simulink model "apf"  (R2025b)
settings: Solver=ode1  StartTime=0.0  StopTime=25  FixedStep=0.05  RelTol=1e-3
libraries: robotcorelib x1
settings Model: Creator=haider  LastModifiedBy=haider

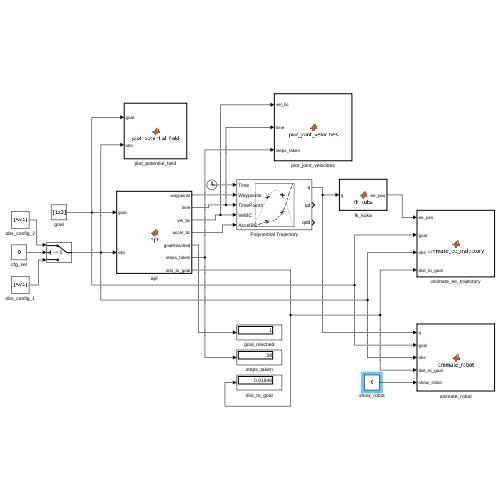
[thumbnail: Simulink's stored preview of the top-level diagram]
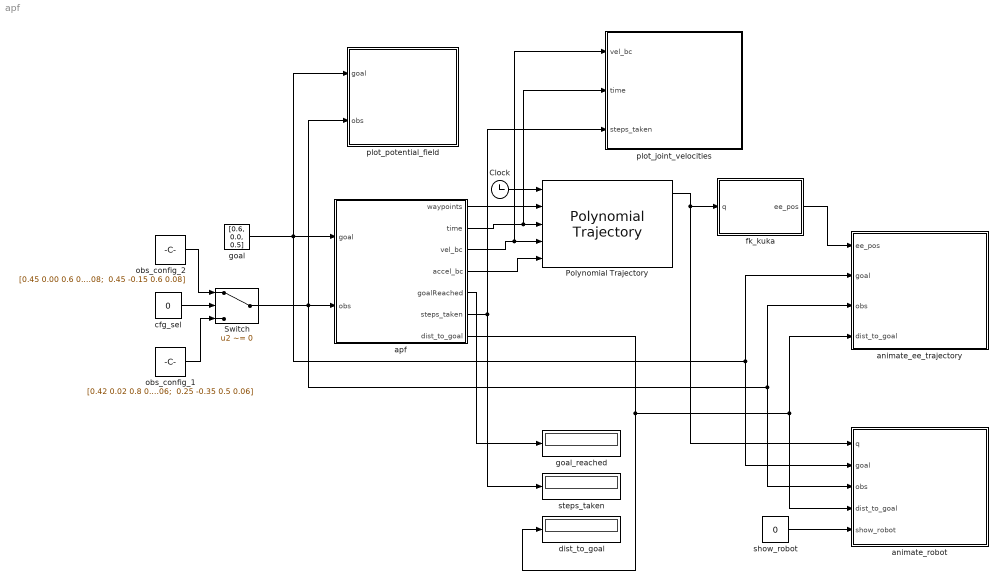
== system apf ==
  Clock : Clock
  Polynomial Trajectory : robotcorelib/Polynomial Trajectory  WaypointSource=External  Waypoints=[ 0, 2, 1, 5, 0; -1, 3, 1, 4, 4 ]  TimePoints=[ 0, 1, 2, 3, 4 ]  TimeInterval=[ 1, 4 ]  Method=Quintic Polynomial  ParameterSource=External  VelocityBoundaryCondition=zeros( 2, 5 )  AccelerationBoundaryCondition=zeros( 2, 5 )  SimulateUsing=Interpreted execution
  Switch : Switch  Criteria=u2 ~= 0  SaturateOnIntegerOverflow=off  InputSameDT=off
  animate_ee_trajectory : MATLAB Function  TreatAsAtomicUnit=on
  animate_robot : MATLAB Function  TreatAsAtomicUnit=on
  apf : MATLAB Function  TreatAsAtomicUnit=on
  cfg_sel : Constant  Value=0
  dist_to_goal : Display
  fk_kuka : MATLAB Function  TreatAsAtomicUnit=on
  goal : Constant  Value=[0.6, 0.0, 0.5]  VectorParams1D=off
  goal_reached : Display
  obs_config_1 : Constant  Value=|  VectorParams1D=off
      | [0.42 0.02 0.8 0.06;
      |  0.45 -0.10 0.4 0.06;
      |  0.35 0.15 0.7 0.06;
      |  0.55 0.30 0.4 0.06;
      |  0.25 -0.35 0.5 0.06]
  obs_config_2 : Constant  Value=|  VectorParams1D=off
      | [0.45 0.00 0.6 0.08;
      |  0.35 0.15 0.6 0.08;
      |  0.45 0.15 0.6 0.08;
      |  0.35 -0.15 0.6 0.08;
      |  0.45 -0.15 0.6 0.08]
  plot_joint_velocities : MATLAB Function  TreatAsAtomicUnit=on
  plot_potential_field : MATLAB Function  TreatAsAtomicUnit=on
  show_robot : Constant  Value=0
  steps_taken : Display
  wires:
  goal/1 -> plot_potential_field/1(goal), animate_robot/2(goal), animate_ee_trajectory/2(goal), apf/1(goal)
  Switch/1 -> animate_robot/3(obs), animate_ee_trajectory/3(obs), plot_potential_field/2(obs), apf/2(obs)
  cfg_sel/1 -> Switch/2
  obs_config_2/1 -> Switch/1
  obs_config_1/1 -> Switch/3
  Clock/1 -> Polynomial Trajectory/1
  apf/1(waypoints) -> Polynomial Trajectory/2
  apf/2(time) -> Polynomial Trajectory/3, plot_joint_velocities/2(time)
  apf/3(vel_bc) -> plot_joint_velocities/1(vel_bc), Polynomial Trajectory/4
  apf/4(accel_bc) -> Polynomial Trajectory/5
  Polynomial Trajectory/1 -> fk_kuka/1(q), animate_robot/1(q)
  fk_kuka/1(ee_pos) -> animate_ee_trajectory/1(ee_pos)
  apf/7(dist_to_goal) -> dist_to_goal/1, animate_robot/4(dist_to_goal), animate_ee_trajectory/4(dist_to_goal)
  show_robot/1 -> animate_robot/5(show_robot)
  apf/6(steps_taken) -> steps_taken/1, plot_joint_velocities/3(steps_taken)
  apf/5(goalReached) -> goal_reached/1

== matlab function apf/plot_potential_field ==
  data: goal input; obs input
function plot_potential_field(goal, obs)
%#codegen

persistent fig_created;

if isempty(fig_created)
    fig_created = false;
end

k_att  = 4.0;
k_rep  = 0.04;
d_star = 0.3;
rho_0  = 0.05;

res     = 100;
x_range = linspace(-0.5, 1.0, res);
y_range = linspace(-0.5, 1.0, res);

z_slice = goal(3);

[X, Y] = meshgrid(x_range, y_range);

U_total = zeros(res, res);

for xi = 1:res
    for yi = 1:res

        p = [X(yi,xi), Y(yi,xi), z_slice];

        % Attractive potential
        rho_att = norm(p - goal);

        if rho_att <= d_star
            U_att = 0.5 * k_att * rho_att^2;
        else
            U_att = d_star * k_att * rho_att ...
                  - 0.5 * k_att * d_star^2;
        end

        % Repulsive potential
        U_rep = 0;

        for j = 1:size(obs,1)

            obs_p = obs(j,1:3);
            obs_r = obs(j,4);

            rho = norm(p - obs_p) - obs_r;

            if rho <= rho_0 && rho > 0.001
                U_rep = U_rep + ...
                    0.5 * k_rep * (1/rho - 1/rho_0)^2;
            end

        end

        U_total(yi,xi) = U_att + U_rep;

    end
end

if ~fig_created

    fig_created = true;

    % Clip extreme values for better visualization
    U_plot = min(U_total, prctile(U_total(:),95));

    figure('Visible','on');

    surf(X,Y,U_plot,'EdgeColor','none');

    colormap(gca,jet);
    colorbar;
    hold on;

    % Goal marker
    plot3(goal(1),goal(2),0,...
        'gp',...
        'MarkerSize',15,...
        'MarkerFaceColor','g');

    % Obstacle slice outlines
    for j = 1:size(obs,1)

        obs_p = obs(j,1:3);
        obs_r = obs(j,4);

        dz = abs(obs_p(3) - z_slice);

        if dz < obs_r

            r_slice = sqrt(obs_r^2 - dz^2);

            theta = linspace(0,2*pi,60);

            cx = obs_p(1) + r_slice*cos(theta);
            cy = obs_p(2) + r_slice*sin(theta);

            plot3(cx,cy,zeros(size(cx)),...
                'r-',...
                'LineWidth',2);

        end

    end

    xlabel('X (m)');
    ylabel('Y (m)');
    zlabel('U_{total}');

    title(sprintf( ...
        'APF Potential Landscape (z = %.2f m)', ...
        z_slice));

    view(45,35);
    grid on;

end

end

== matlab function apf/apf ==
  data: goal input; waypoints output; obs input; time output; vel_bc output; accel_bc output; goalReached output; steps_taken output; dist_to_goal output
function [waypoints, time, vel_bc, accel_bc, goalReached, steps_taken, dist_to_goal] = apf(goal, obs)

%#codegen
MAX_ITER = 500;


persistent planned

persistent wp_cache
persistent time_cache
persistent vel_cache
persistent accel_cache
persistent goal_cache
persistent steps_cache
persistent dist_cache

if isempty(planned)

    planned = false;

    wp_cache    = zeros(7,MAX_ITER);
    time_cache  = zeros(1,MAX_ITER);
    vel_cache   = zeros(7,MAX_ITER);
    accel_cache = zeros(7,MAX_ITER);

    goal_cache  = false;
    steps_cache = int32(0);
    dist_cache  = 0;

end

if planned

    waypoints    = wp_cache;
    time         = time_cache;
    vel_bc       = vel_cache;
    accel_bc     = accel_cache;
    goalReached  = goal_cache;
    steps_taken  = steps_cache;
    dist_to_goal = dist_cache;

    return;

end


% Pre-allocate fixed-size outputs with NaN so unused slots are ignored
waypoints = nan(7, MAX_ITER);
vel_bc    = nan(7, MAX_ITER);
accel_bc  = nan(7, MAX_ITER);
time      = zeros(1, MAX_ITER);

goalReached = false;
steps_taken = int32(0);

% APF params
k_att     = 4.0;
k_rep     = 0.04;
dt        = 0.05;
threshold = 0.02;
rho_0     = 0.05;
iterations = MAX_ITER;
d_star    = 0.3;
q_dot_max = 5.0;

ee_body = 'iiwa_link_ee';

collision_links = { ...
    'iiwa_link_4'; ...
    'iiwa_link_5'; ...
    'iiwa_link_6'; ...
    'iiwa_link_ee' ...
};

robot = loadrobot('kukaIiwa14', 'DataFormat', 'row');
q = homeConfiguration(robot);   % 1x7 row vector

goal = goal(:)';

pos_buffer = zeros(3, 15);
q_dot_prev = zeros(1,7);

for i = 1:iterations

    % Forward kinematics
    T_ee = getTransform(robot, q, ee_body);
    x_ee = T_ee(1:3, 4)';    % 1x3

    % Error to goal
    dx = x_ee - goal;
    dist_to_goal = norm(dx);

    % Convergence check
    if dist_to_goal < threshold
        goalReached = true;
        steps_taken = int32(i);
        break;
    end

    % A. Attractive force
    if dist_to_goal <= d_star
        F_att = -k_att * dx;    % quadratic
    else
        F_att = -d_star * k_att * (dx / dist_to_goal);   % conic
    end

    % EE Jacobian — fixed-size copy for codegen stability
    J_tmp = geometricJacobian(robot, q, ee_body);

    J_ee = zeros(6,7);
    J_ee(:,:) = J_tmp;

    % Attractive joint velocity (pseudo-inverse of 3x7 linear part)
    q_dot_total = (pinv(J_ee(4:6,:)) * F_att')';   % 1x7

    % B. Repulsive forces (all collision links + all obstacles)
    F_rep_total = zeros(1,3);
    for L = 1:4
    
        link_name = collision_links{L};
    
        T_link = getTransform(robot, q, link_name);
        x_link = T_link(1:3,4)';
    
        for j = 1:size(obs,1)
    
            obs_p = obs(j,1:3);
            obs_r = obs(j,4);
    
            dist_vec = x_link - obs_p;
            dist_to_center = norm(dist_vec);
    
            rho = dist_to_center - obs_r;
    
            if rho <= rho_0 && rho > 0.001
    
                rep_mag = k_rep * ...
                    (1/rho - 1/rho_0) * ...
                    (1/rho^2);
    
                F_rep_total = F_rep_total + ...
                    rep_mag * (dist_vec / dist_to_center);
    
            end
    
        end
    
        J_tmp2 = geometricJacobian(robot,q,link_name);
    
        J_link = zeros(6,7);
        J_link(:,:) = J_tmp2;
    
        q_dot_link = (pinv(J_link(4:6,:)) * F_rep_total')';
    
        q_dot_total = q_dot_total + q_dot_link;
    
    end

    F_total = F_att + F_rep_total;

    stuck = false;

    % Case 1 — absolute local minimum
    if norm(F_total) < 1e-3 && dist_to_goal > threshold
        stuck = true;
    end

    % Case 2 — limit cycle / oscillation
    pos_buffer(:, mod(i-1, 15)+1) = x_ee';

    if i > 15

        old_idx = mod(i-15, 15) + 1;

        if norm(x_ee' - pos_buffer(:, old_idx)) < 0.01
            stuck = true;
        end
    end

    % Random perturbation
    if stuck
        q = q + (rand(1,7) - 0.5) * 5.0;
        continue;   % skip recording this step
    end

    % Velocity clamp
    max_qdot = max(abs(q_dot_total));

    if max_qdot > q_dot_max
        q_dot_total = q_dot_total * (q_dot_max / max_qdot);
    end

    vel_bc(:, i) = q_dot_total';

    if i == 1
        accel_bc(:, i) = zeros(7,1);
    else
        accel_bc(:, i) = (q_dot_total - q_dot_prev)' / dt;
    end

    q_dot_prev = q_dot_total;

    waypoints(:, i) = q';

    q = q + q_dot_total * dt;

    steps_taken = int32(i);

end

% APF loop
valid = all(~isnan(waypoints),1);
m = sum(valid);

if m > 0

    waypoints(:,1:m) = waypoints(:,valid);
    vel_bc(:,1:m) = vel_bc(:,valid);
    accel_bc(:,1:m) = accel_bc(:,valid);

    if m < MAX_ITER

        last_q = waypoints(:,m);
        last_v = vel_bc(:,m);
        last_a = accel_bc(:,m);

        waypoints(:,m+1:end) = repmat(last_q,1,MAX_ITER-m);
        vel_bc(:,m+1:end) = repmat(last_v,1,MAX_ITER-m);
        accel_bc(:,m+1:end) = repmat(last_a,1,MAX_ITER-m);

    end

    time = (0:MAX_ITER-1) * dt;

    steps_taken = int32(m);

end

wp_cache     = waypoints;
time_cache   = time;
vel_cache    = vel_bc;
accel_cache  = accel_bc;
goal_cache   = goalReached;
steps_cache  = steps_taken;
dist_cache   = dist_to_goal;

planned = true;

end

== matlab function apf/fk_kuka ==
  data: q input; ee_pos output
function ee_pos = fk_kuka(q)

persistent robot

if isempty(robot)
    robot = loadrobot('kukaIiwa14','DataFormat','row');
end

% Convert 7x1 -> 1x7
q = q(:)';

T = getTransform(robot, q, 'iiwa_link_ee');

ee_pos = T(1:3,4);

end

== matlab function apf/animate_ee_trajectory ==
  data: ee_pos input; goal input; obs input; dist_to_goal input
function animate_ee_trajectory(ee_pos, goal, obs, dist_to_goal)

%#codegen

coder.extrinsic( ...
    'figure','axes','hold','grid','axis','view', ...
    'plot3','surf','set','drawnow','title');

persistent fig ax path sx sy sz
persistent trace_xs trace_ys trace_zs idx

if isempty(fig)

    trace_xs = nan(1,5000);
    trace_ys = nan(1,5000);
    trace_zs = nan(1,5000);

    idx = int32(0);

    fig = figure('Name','EE Trajectory');
    ax = axes('Parent',fig);

    hold(ax,'on');
    grid(ax,'on');
    axis(ax,'equal');

    view(ax,140,20);
    axis(ax,[-0.5 1 -0.5 1 0 1.2]);

    plot3(ax, goal(1), goal(2), goal(3), 'gs', 'MarkerSize', 12, 'LineWidth', 2);

    u = linspace(0,2*pi,17);
    v = linspace(0,pi,17);

    sx = zeros(17,17);
    sy = zeros(17,17);
    sz = zeros(17,17);

    for i = 1:17
        for j = 1:17

            sx(i,j) = cos(u(i))*sin(v(j));
            sy(i,j) = sin(u(i))*sin(v(j));
            sz(i,j) = cos(v(j));

        end
    end

    for k = 1:size(obs,1)

        o = obs(k,:);

        surf( ...
            ax, ...
            sx*o(4)+o(1), ...
            sy*o(4)+o(2), ...
            sz*o(4)+o(3), ...
            'FaceAlpha',0.5, ...
            'EdgeColor','none');

    end

    path = plot3( ...
        ax, ...
        nan,nan,nan, ...
        'b-', ...
        'LineWidth',2);

    drawnow;

end

if any(isnan(ee_pos))
    return;
end

idx = idx + 1;

trace_xs(idx) = ee_pos(1);
trace_ys(idx) = ee_pos(2);
trace_zs(idx) = ee_pos(3);

valid = ~isnan(trace_xs);

set(path, ...
    'XData',trace_xs(valid), ...
    'YData',trace_ys(valid), ...
    'ZData',trace_zs(valid));

title(ax, sprintf('Dist. to goal: %.4f', dist_to_goal));

drawnow limitrate;

end

== matlab function apf/animate_robot ==
  data: q input; goal input; obs input; dist_to_goal input; show_robot input
function animate_robot(q, goal, obs, dist_to_goal, show_robot)
%#codegen

coder.extrinsic('figure','axes','hold','grid','axis','view', ...
'xlabel','ylabel','zlabel','title','plot3','surf', ...
'set','drawnow','loadrobot','show','getTransform')

% -----------------------
% HARD DISABLE VISUALIZATION
% -----------------------
if show_robot == 0
    return;
end

persistent fig ax path robot trace_xs trace_ys trace_zs sx sy sz idx

if isempty(fig)

robot = loadrobot('kukaIiwa14','DataFormat','row');

trace_xs = nan(1,500);
trace_ys = nan(1,500);
trace_zs = nan(1,500);
idx = int32(0);

fig = figure('Name','APF');
ax = axes('Parent',fig);
hold(ax,'on'); grid(ax,'on');
axis(ax,'equal');
view(ax,140,20);
axis(ax,[-0.5 1 -0.5 1 0 1.2]);

plot3(ax, goal(1), goal(2), goal(3), 'gs', 'MarkerSize', 12, 'LineWidth', 2);

u = linspace(0,2*pi,17);
v = linspace(0,pi,17);

sx = zeros(17,17);
sy = zeros(17,17);
sz = zeros(17,17);

for i=1:17
for j=1:17
sx(i,j)=cos(u(i))*sin(v(j));
sy(i,j)=sin(u(i))*sin(v(j));
sz(i,j)=cos(v(j));
end
end

n_obs = size(obs,1);
for j=1:n_obs
o = obs(j,:);
surf(ax,sx*o(4)+o(1),sy*o(4)+o(2),sz*o(4)+o(3), ...
'FaceAlpha',0.5,'EdgeColor','none');
end

path = plot3(ax,nan,nan,nan,'b-','LineWidth',2);

drawnow;
end

% -----------------------
% safety
% -----------------------
if any(isnan(q))
return;
end

% force correct shape (CRITICAL)
q = q(:)';

% -----------------------
% update index
% -----------------------
idx = idx + 1;
if idx > 500
    idx = int32(1);
end

% -----------------------
% FK
% -----------------------
T_tmp = getTransform(robot,q,'iiwa_link_ee');

T = zeros(4,4);
T(:,:) = T_tmp;

p = zeros(1,3);
p(1) = T(1,4);
p(2) = T(2,4);
p(3) = T(3,4);

trace_xs(idx)=p(1);
trace_ys(idx)=p(2);
trace_zs(idx)=p(3);

valid = ~isnan(trace_xs);

set(path, ...
'XData',trace_xs(valid), ...
'YData',trace_ys(valid), ...
'ZData',trace_zs(valid));

% -----------------------
% robot render (optional)
% -----------------------
if show_robot
    show(robot, q, ...
        'Parent',ax, ...
        'PreservePlot',false, ...
        'Frames','off');
end

% -----------------------
% UI
% -----------------------

title(ax,sprintf('Dist. to goal: %.4f', dist_to_goal));

drawnow limitrate;

end

== matlab function apf/plot_joint_velocities ==
  data: vel_bc input; time input; steps_taken input
function plot_joint_velocities(vel_bc, time, steps_taken)
%#codegen

coder.extrinsic('figure','plot','xlabel','ylabel', ...
                'title','legend','grid','hold')

persistent plotted

if isempty(plotted)
    plotted = false;
end

% Plot only once
if plotted
    return;
end

N = double(steps_taken);

if N <= 1
    return;
end

figure('Name','Joint Velocity Profiles');

plot(time(1:N), vel_bc(:,1:N)');

xlabel('Time (s)');
ylabel('Joint Velocity (rad/s)');
title('Joint Velocity Profiles');

legend('J1','J2','J3','J4','J5','J6','J7');

grid on;

plotted = true;

end
